simulink model "simu_practica7"  (R2023b)
settings: Solver=VariableStepAuto  StartTime=0.0  StopTime=10.0  RelTol=1e-3
values from neighbouring files (symbols this model uses):
  Capacitor1 = 100e-9    (= 1e-07)    [CFRO.m]    (also in Parametros_practica_7.m)
  Capacitor2 = 100e-9    (= 1e-07)    [CFRO.m]    (also in Parametros_practica_7.m)
  Resistencia1 = 5e6    (= 5000000)    [CFRO.m]    (also in Parametros_practica_7.m)
  Resistencia2 = 5e6    (= 5000000)    [CFRO.m]    (also in Parametros_practica_7.m)
  Resistencia3 = 5e6    (= 5000000)    [CFRO.m]    (also in Parametros_practica_7.m)
settings Model: Creator=mluser  LastModifiedBy=mluser

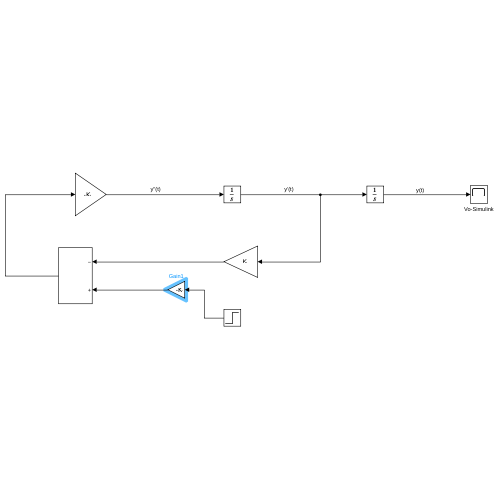
[thumbnail: Simulink's stored preview of the top-level diagram]
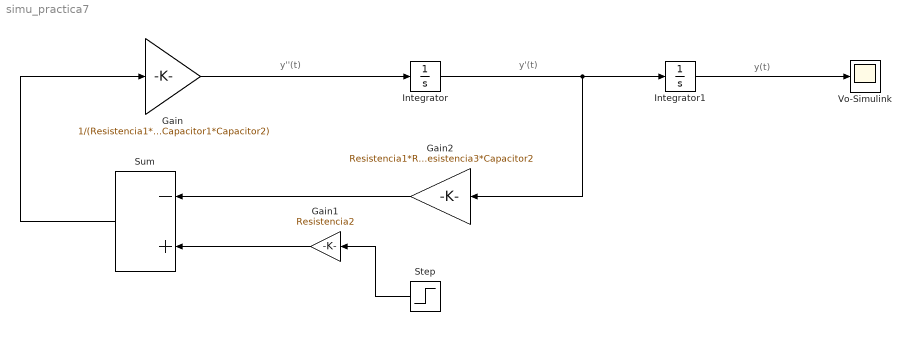
== system simu_practica7 ==
  note: y(t)
  note: y'(t)
  note: y''(t)
  Gain : Gain  Gain=1/(Resistencia1*Resistencia2*Resistencia3*Capacitor1*Capacitor2)
  Gain1 : Gain  Gain=Resistencia2
  Gain2 : Gain  Gain=Resistencia1*Resistencia3*Capacitor2
  Integrator : Integrator
  Integrator1 : Integrator
  Step : Step  Time=0  SampleTime=0
  Sum : Sum  Inputs=-+
  Vo-Simulink : Scope
  wires:
  Gain/1 -> Integrator/1
  Sum/1 -> Gain/1
  Integrator/1 -> Gain2/1, Integrator1/1
  Step/1 -> Gain1/1
  Integrator1/1 -> Vo-Simulink/1
  Gain1/1 -> Sum/2
  Gain2/1 -> Sum/1
